simulink model "hdlconvert_tb"  (R2019b)
settings: Solver=VariableStepAuto  StartTime=0.0  StopTime=3* 2^8  RelTol=1e-3  EnableMultiTasking=on
libraries: lib_dsphdltypes_v1 x6, simulink x1, dspsrcs4 x1
settings Model: Creator=babstm  LastModifiedBy=mbabst
settings DataIOCC: LimitDataPoints=on  ReturnWorkspaceOutputs=off
settings OptimizationCC: BlockReduction=off  ConditionallyExecuteInputs=off  DefaultParameterBehavior=Inlined  LifeSpan=inf
settings DebuggingCC: AlgebraicLoopMsg=error  AllowSymbolicDim=off  SFUnexpectedBacktrackingDiag=warning  SFNoUnconditionalDefaultTransitionDiag=warning  SFExecutionAtInitializationDiag=none  ArithmeticOperatorsInVariantConditions=warning
settings HardwareCC: ProdBitPerPointer=32  ProdBitPerSizeT=32  ProdBitPerPtrDiffT=32  ProdLargestAtomicFloat=None  ProdIntDivRoundTo=Undefined  ProdEndianess=Unspecified  ProdWordSize=32  ProdHWDeviceType=ASIC/FPGA->ASIC/FPGA  ProdEqTarget=off
settings ModelReferenceCC: PropagateSignalLabelsOutOfModel=off
settings SFSimCC: SimUseLocalCustomCode=off  CustomCodeUndefinedFunction=UseInterfaceOnly
settings RTWCC: RTWUseLocalCustomCode=off
settings CodeAppCC: StateflowObjectComments=on
settings GRTTargetCC: TargetLangStandard=C89/C90 (ANSI)
settings ConfigComp: CovMetricSettings=dw  CovHtmlReporting=on  CovSaveCumulativeToWorkspaceVar=on  CovSaveSingleToWorkspaceVar=on  CovExternalEMLEnable=off

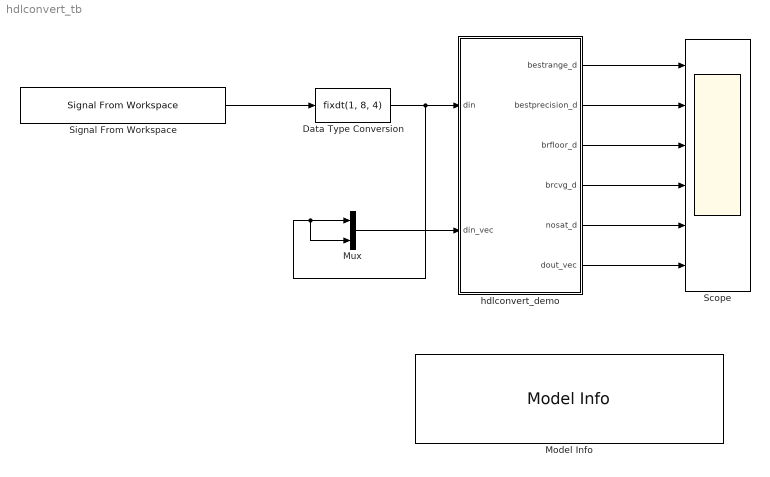
== system hdlconvert_tb ==
  Data Type Conversion : DataTypeConversion  OutDataTypeStr=fixdt(1, 8, 4)  ConvertRealWorld=Stored Integer (SI)
  Model Info : simulink/Model-Wide Utilities/Model Info  Frame=on  DisplayStringWithTags=|  HorizontalTextAlignment=Left  LeftAlignmentValue=0.02
      | Copyright (c) 2005-2021 DSPlogic, Inc.
      | Distributed under the terms of the Simplified BSD License.
      | The full license is in the file LICENSE, distributed with this software.
      | 
      | Model: %<ModelName> (v%<ModelVersion>)
      | Author: Michael Babst <mike.babst@dsplogic.com>
      | Created: by %<Creator> on %<Created>
      | Modified: by %<ModifiedBy> on %<LastModificationDate>
  Mux : Mux  Inputs=2
  Scope : Scope  NumInputPorts=6
  Signal From Workspace : dspsrcs4/Signal From Workspace  X=[(0:2^7-1) (2^7-1-2:-1:-2^7 ) (-2^7 : -1) ]  Ts=1  nsamps=1  OutputAfterFinalValue=Cyclic repetition  ignoreOrWarnInputAndFrameLengths=on  OutputFrames=off
  hdlconvert_demo : Subsystem
  wires:
  Signal From Workspace/1 -> Data Type Conversion/1
  Data Type Conversion/1 -> Mux/2, Mux/1, hdlconvert_demo/1(din)
  Mux/1 -> hdlconvert_demo/2(din_vec)
  hdlconvert_demo/1(bestrange_d) -> Scope/1
  hdlconvert_demo/2(bestprecision_d) -> Scope/2
  hdlconvert_demo/3(brfloor_d) -> Scope/3
  hdlconvert_demo/4(brcvg_d) -> Scope/4
  hdlconvert_demo/5(nosat_d) -> Scope/5
  hdlconvert_demo/6(dout_vec) -> Scope/6

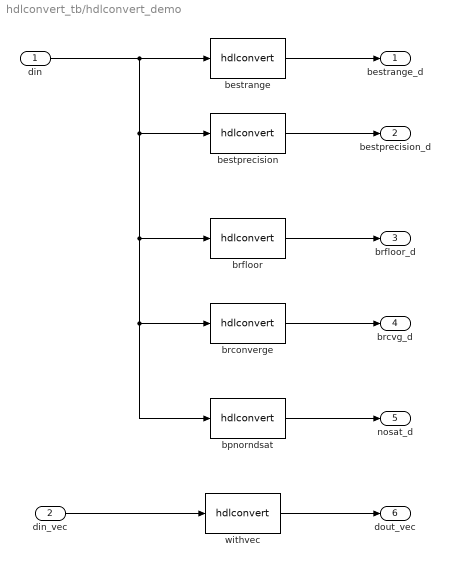
== system hdlconvert_tb/hdlconvert_demo ==
  din : Inport
  din_vec : Inport  Port=2
  bestprecision : lib_dsphdltypes_v1/hdlconvert  signed=Inherit  maxwidth=6  extend=on  scaleopt=Best Precision  Sforce=0  roundMode=Nearest  saturate=on
      settings: SourceProductName=DSPHDL Library
  bestrange : lib_dsphdltypes_v1/hdlconvert  signed=Inherit  maxwidth=6  extend=on  scaleopt=Best Range  Sforce=0  roundMode=Nearest  saturate=on
      settings: SourceProductName=DSPHDL Library
  bpnorndsat : lib_dsphdltypes_v1/hdlconvert  signed=Inherit  maxwidth=6  extend=on  scaleopt=Best Precision  Sforce=0  roundMode=Floor  saturate=off
      settings: SourceProductName=DSPHDL Library
  brconverge : lib_dsphdltypes_v1/hdlconvert  signed=Inherit  maxwidth=6  extend=on  scaleopt=Best Range  Sforce=0  roundMode=Convergent  saturate=on
      settings: SourceProductName=DSPHDL Library
  brfloor : lib_dsphdltypes_v1/hdlconvert  signed=Inherit  maxwidth=6  extend=on  scaleopt=Best Range  Sforce=0  roundMode=Floor  saturate=on
      settings: SourceProductName=DSPHDL Library
  withvec : lib_dsphdltypes_v1/hdlconvert  signed=Inherit  maxwidth=6  extend=on  scaleopt=Best Precision  Sforce=0  roundMode=Floor  saturate=off
      settings: SourceProductName=DSPHDL Library
  bestrange_d : Outport
  bestprecision_d : Outport  Port=2
  brfloor_d : Outport  Port=3
  brcvg_d : Outport  Port=4
  nosat_d : Outport  Port=5
  dout_vec : Outport  Port=6
  wires:
  din/1 -> bestrange/1, brfloor/1, bpnorndsat/1, brconverge/1, bestprecision/1
  bestrange/1 -> bestrange_d/1
  din_vec/1 -> withvec/1
  withvec/1 -> dout_vec/1
  bestprecision/1 -> bestprecision_d/1
  brfloor/1 -> brfloor_d/1
  brconverge/1 -> brcvg_d/1
  bpnorndsat/1 -> nosat_d/1
